simulink model "asbhl20"  (R2016b)
settings: Solver=ode3  StartTime=0.0  StopTime=61  FixedStep=1/120  RelTol=1e-3  AbsTol=1e-6
PreLoadFcn:
  | load asbhl20data.mat
InitFcn:
  | timeSince1970.Value = etime(datevec(now),[1970, 1, 1, 0, 0, 0]);
values from neighbouring files (symbols this model uses):
  maxPackets = 100    [asbhl20data.mat]
  Tc = 0.0166666666667    [asbhl20GlobalChildrenData.mat]
  x_cg = 4.78635044684    [asbhl20data.mat]
undefined symbols (not defined in the file or in its folder): m, message, Receive, s, Send, sigbuilder_block
libraries: aerolibfltsims x5, simulink x4, asbhl20GPS x2, aerolibnav x2, asbhl20env x1, asbhl20airdata x1, asbhl20ralt x1, asbhl20commsys x1, asbhl20FADEC x1, asbhl20sensors x1, asbhl20LGC x1, asbhl20vehicle x1
(part 1 of 3)
Description:
  | HL-20 auto-landing example - top level model / entry point of model
  | 
  | The HL-20 escape vehicle project for the International Space Station was
  | a fully-funded research project, designed at NASA Langley by Bruce
  | Jackson et al. Wind tunnel testing was performed on this design at
  | subsonic, supersonic, and hypersonic conditions on scale models of
  | the prototype concept.
settings Model: FPTRunName=Active  ExtModeTrigMode=oneshot  ExtModeArmWhenConnect=off  ExtModeAutoUpdateStatusClock=off  Creator=The MathWorks, Inc.  LastModifiedBy=The MathWorks, Inc.
settings SolverCC: ZeroCrossControl=DisableAll
settings DataIOCC: SaveFormat=StructureWithTime  SaveOutput=off  SignalLogging=off  SaveTime=off  StateSaveName=xbase  TimeSaveName=tsim  OutputSaveName=ysim  SignalLoggingName=sigsOut
settings OptimizationCC: BlockReduction=off  OptimizeBlockIOStorage=off  BufferReuse=off  GlobalBufferReuse=off  ExpressionFolding=off  ExpressionDepthLimit=2147483647  LocalBlockOutputs=off  InitFltsAndDblsToZero=on  EfficientFloat2IntCast=on  LifeSpan=inf
settings DebuggingCC: UnderspecifiedInitializationDetection=Classic  CheckExecutionContextPreStartOutputMsg=on  CheckExecutionContextRuntimeOutputMsg=on  MultiTaskCondExecSysMsg=none  SigSpecEnsureSampleTimeMsg=none  ParameterPrecisionLossMsg=none  FcnCallInpInsideContextMsg=warning  UniqueDataStoreMsg=error  AllowSymbolicDim=off  ModelReferenceSymbolNameMessage=none  StateNameClashWarn=warning  StrictBusMsg=ErrorOnBusTreatedAsVector  SFUnexpectedBacktrackingDiag=warning  SFNoUnconditionalDefaultTransitionDiag=warning  SFExecutionAtInitializationDiag=none
settings HardwareCC: ProdBitPerPointer=32  ProdBitPerSizeT=32  ProdBitPerPtrDiffT=32  ProdLargestAtomicFloat=None  ProdIntDivRoundTo=Undefined  ProdEndianess=Unspecified  ProdWordSize=32  ProdHWDeviceType=32-bit Generic  TargetBitPerPointer=64  TargetBitPerSizeT=64  TargetBitPerPtrDiffT=64  TargetLongLongMode=on  TargetIntDivRoundTo=Zero  TargetEndianess=LittleEndian  TargetWordSize=64  TargetHWDeviceType=MATLAB Host
settings ModelReferenceCC: UpdateModelReferenceTargets=IfOutOfDate  CheckModelReferenceTargetMessage=none  ModelReferencePassRootInputsByReference=off  PropagateSignalLabelsOutOfModel=off
settings SFSimCC: SimParseCustomCode=off
settings CodeAppCC: MaxIdLength=63
settings GRTTargetCC: TargetLangStandard=C89/C90 (ANSI)  GeneratePreprocessorConditionals=Disable all  CombineOutputUpdateFcns=off  GRTInterface=on
settings ConfigComp: CovMetricSettings=d  CovHtmlReporting=on  CovSaveCumulativeToWorkspaceVar=on  CovSaveSingleToWorkspaceVar=on  CovExternalEMLEnable=off  CovSFcnEnable=off

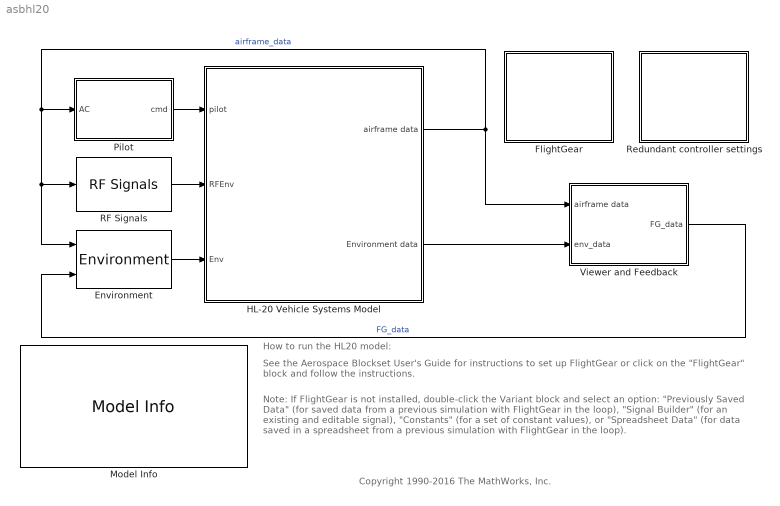
== system asbhl20 ==
  note: Copyright 1990-2016 The MathWorks, Inc.
  note: How to run the HL20 model:
  note: See the Aerospace Blockset User's Guide for instructions to set up FlightGear or click on the "FlightGear" block and follow the instructions.
  note: Note: If FlightGear is not installed, double-click the Variant block and select an option: "Previously Saved Data" (for saved data from a previous simulation with FlightGear in the loop), "Signal Builder" (for an existing and editable signal), "Constants" (for a set of constant values), or "Spreadsheet Data" (for data saved in a spreadsheet from a previous simulation with FlightGear in the loop).
  Environment : asbhl20env/Environment  SystemSampleTime=-1
  FlightGear : Subsystem  mask(FlightGear){baseFG=C:\Program Files\FlightGear\}
      mask prompts: baseFG "2. Specify FlightGear base directory"
      mask help:
      | To run this example using FlightGear locally:
      |
      | 1. Download and install FlightGear. This action opens the FlightGear download page. From this page, download and install FlightGear.
      |
      | 2. Specify FlightGear base directory.
      |
      | 3. Check FlightGear base directory. Click this button to check that FlightGear is correctly configured and installed. Upon success, the Run FlightGear block turns green and the text changes to "Start FlightGear".
      |
      | 4. Launch FlightGear for HL-20. This button installs HL-20 and runs FlightGear.
      |
      | Note: You may need administrator privilege to install HL-20.
      mask init:
      | mdl = gcs;
      | blk = gcb;
      | asbCopyAndStartFlightGear(blk,mdl,'Check','init');
      settings: AttributesFormatString=Install FlightGear
      mask Help: helpview([docroot,'/toolbox/aeroblks/aeroblks.map'],'hl20_flight_gear_help')
      mask DialogControl installFG Prompt: 1. Download and Install FlightGear
      mask DialogControl installFG Callback: web('http://flightgear.org/download/','-browser')
      mask DialogControl updateFG Prompt: 3. Check Base Directory
      mask DialogControl updateFG Callback: asbCopyAndStartFlightGear(gcb,gcs,'Check','button');
      mask DialogControl launchFG Prompt: 4. Launch HL-20 in FlightGear
      mask DialogControl launchFG Callback: asbCopyAndStartFlightGear(gcb,gcs,'CopyStart')
      mask Display: image('asbHL20FGLanding.png',[.1, .1, .8, .8],'on');
  HL-20 Vehicle Systems Model : Subsystem
      settings: RTWSystemCode=Inline
      mask Display: image('asbHL20pic.jpg')
  Model Info : simulink/Model-Wide Utilities/Model Info  BlockCM=none  Frame=on  DisplayStringWithTags=|  HorizontalTextAlignment=Center  LeftAlignmentValue=0.5  SourceBlockDiagram=asbhl20  TagMaxNumber=20
      | HL-20 Example,
      | version %<ModelVersion>
      | Aerodynamic model from 
      | Jackson E. B., Cruz C. L., 
      | "Preliminary Subsonic Aerodynamic
      | Model for Simulation Studies of the
      | HL-20 Lifting Body", 
      | NASA TM4302, August 1992.
  Pilot : Subsystem  TreatAsAtomicUnit=on
  RF Signals : asbhl20RF/RF Signals
  Redundant controller settings : Subsystem  mask(Select Redundant Controller){}
      mask help:
      | This model has a reactive controller that uses a fault-tolerant design. The controller modifies the actuator and hydraulic system as necessary. It uses a specifically designed mode logic.
      |
      | Select the implementation mode logic of the controller. The mode logic determines the actuator setup in the event of a hydraulic or actuator failure.
      |
      | Open the failure insertion panel to simulate hydraulic or actuator failures.
      |
      | Note: This feature requires a Stateflow license.
      mask init:
      | installedProducts = ver;
      | stateflowFlag = false;
      | for k=1:length(installedProducts)
      |     if strcmp(installedProducts(k).Name,'Stateflow')
      |         testLicense = license('test','stateflow');
      |         if testLicense
      |             stateflowFlag = true;
      |         end
      |     end
      | end
      | MaskObject = get_param(gcb,'MaskObject');
      | sfButtonObject = MaskObject.getDialogControl('sfLogic');
      | ssButtonObject = MaskObject.getDialogControl('ssLogic');
      | mrButtonObject = MaskObject.getDialogControl('mrLogic');
      | omButtonObject = MaskObject.getDialogControl('openModeLogic');
      | fButtonObject = MaskObject.getDialogControl('failButton');
      | if stateflowFlag
      |     sfButtonObject.Enabled = 'on';
      |     ssButtonObject.Enabled = 'on';
      |     mrButtonObject.Enabled = 'on';
      |     omButtonObject.Enabled = 'on';
      |     fButtonObject.Enabled = 'on';
      | else
      |     sfButtonObject.Enabled = 'off';
      |     ssButtonObject.Enabled = 'off';
      |     mrButtonObject.Enabled = 'off';
      |     omButtonObject.Enabled = 'off';
      |     fButtonObject.Enabled = 'off';
      | end
      | sfVar = evalin('base','Variants.FDIRApp');
      | switch sfVar
      |     case 0
      |         attStr = 'No Mode Logic';
      |     case 1
      |         attStr = 'Stateflow Chart in Subsystem';
      |     case 2
      |         attStr = 'Stateflow Chart in Model';
      |     case 3
      |         attStr = 'Stateflow Chart';
      | end
      | sfVarCheck = get_param(gcb,'AttributesFormatString');
      | if ~strcmp(sfVarCheck,attStr)
      |     set_param(gcb,'AttributesFormatString',attStr);
      | end
      settings: AttributesFormatString=No Mode Logic
      mask Help: web('http://www.mathworks.com/tagteam/21848_Mosterman Ghidella AIAA 2004 Final.pdf','-browser');
      mask DialogControl failButton Prompt: Open Failure Insertion Panel
      mask DialogControl failButton Callback: open_system(sprintf(['asbhl20/HL-20 Vehicle Systems Model/Avionics/Actuator \nSystem Failures ']),'window');
      mask DialogControl openModeLogic Prompt: Open Mode Logic
      mask DialogControl openModeLogic Callback:
      | load_system('asbhl20_FDIRApp');
      | varLogic = evalin('base','Variants.FDIRApp');
      | switch varLogic
      |     case 0
      |         open_system('asbhl20_FDIRApp/Mode Logic for Wing, Upper, and Lower/Variant Subsystem/No Logic');
      |     case 1
      |         open_system('asbhl20_FDIRApp/Mode Logic for Wing, Upper, and Lower/Variant Subsystem/Mode Logic SS/Mode Logic Chart');
      |     case 2
      |         open_system('asbhl20_FDIRApp/Mode Logic for Wing, Upper, and Lower/Variant Subsystem/Mode Logic App/Mode Logic App');
      |         open_system('asbhl20_FDIRmodelogicApp/Mode Logic');
      |     case 3
      |         open_system('asbhl20_FDIRApp/Mode Logic for Wing, Upper, and Lower/Variant Subsystem/Mode Logic Chart');
      | end
      mask DialogControl paper Prompt: Model Reuse for the Training of Fault Scenarios in Aerospace
      mask DialogControl paper Callback: web('http://www.mathworks.com/tagteam/21848_Mosterman Ghidella AIAA 2004 Final.pdf','-browser');
      mask Display: image('asbHL20ActuatorRedundancy.svg')
  Viewer and Feedback : Subsystem  Variant=on  mask(Closed Loop Variant System){}
      mask help: Select a simulation variant to identify the data source. For example, for batch mode select either a Signal Builder block or a previously saved data file. If your data source is FlightGear, run the simulation in Normal mode.
      settings: AttributesFormatString=%<ActiveVariant>
  wires:
  HL-20 Vehicle Systems Model/1(airframe data) -> Pilot/1(AC), RF Signals/1, Environment/1, Viewer and Feedback/1(airframe data)  "airframe_data"
  Pilot/1(cmd) -> HL-20 Vehicle Systems Model/1(pilot)
  Environment/1 -> HL-20 Vehicle Systems Model/3(Env)
  RF Signals/1 -> HL-20 Vehicle Systems Model/2(RFEnv)
  HL-20 Vehicle Systems Model/2(Environment data) -> Viewer and Feedback/2(env_data)
  Viewer and Feedback/1(FG_data) -> Environment/2  "FG_data"

== system asbhl20/FlightGear ==

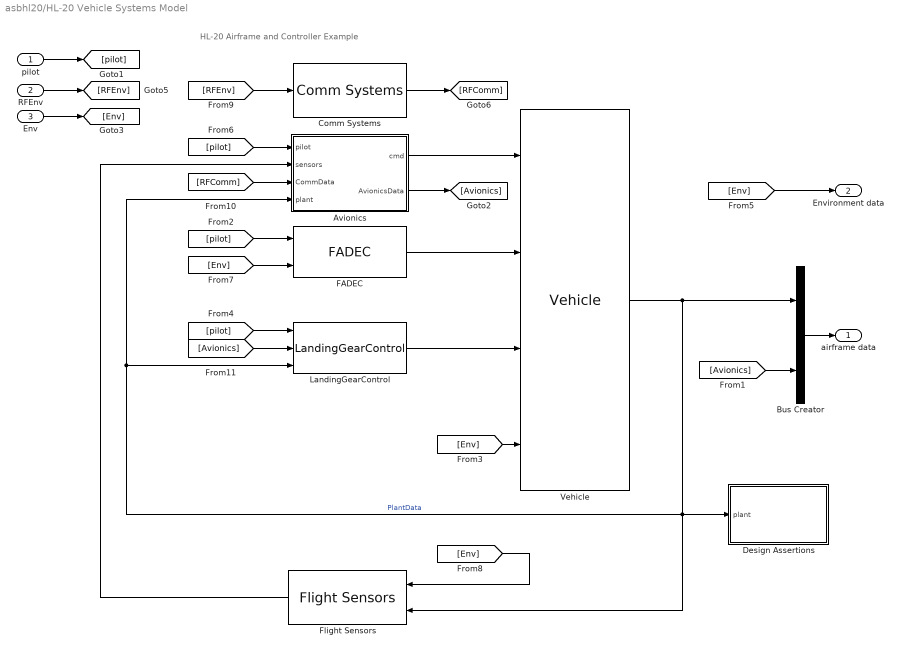
== system asbhl20/HL-20 Vehicle Systems Model ==
  note: HL-20 Airframe and Controller Example
  pilot : Inport
  RFEnv : Inport  Port=2
  Env : Inport  Port=3
  Avionics : Subsystem
  Bus Creator : BusCreator  Inputs=2
  Comm Systems : asbhl20commsys/Comm Systems
  Design Assertions : Subsystem
  FADEC : asbhl20FADEC/FADEC
  Flight Sensors : asbhl20sensors/Flight Sensors
  LandingGearControl : asbhl20LGC/LandingGearControl
  Vehicle : asbhl20vehicle/Vehicle
  airframe data : Outport
  Environment data : Outport  Port=2
  wires:
  [Env] -> Environment data/1
  [Avionics] -> LandingGearControl/2
  Avionics/1(cmd) -> Vehicle/1
  Avionics/2(AvionicsData) -> [Avionics]
  [RFComm] -> Avionics/3(CommData)
  [RFEnv] -> Comm Systems/1
  Comm Systems/1 -> [RFComm]
  [Env] -> Flight Sensors/1
  RFEnv/1 -> [RFEnv]
  Flight Sensors/1 -> Avionics/2(sensors)
  [Env] -> FADEC/2
  [pilot] -> Avionics/1(pilot)
  pilot/1 -> [pilot]
  [pilot] -> LandingGearControl/1
  [pilot] -> FADEC/1
  [Env] -> Vehicle/4
  Env/1 -> [Env]
  LandingGearControl/1 -> Vehicle/3
  FADEC/1 -> Vehicle/2
  Bus Creator/1 -> airframe data/1
  [Avionics] -> Bus Creator/2
  Vehicle/1 -> Flight Sensors/2, LandingGearControl/3, Avionics/4(plant), Design Assertions/1(plant), Bus Creator/1  "PlantData"

== system asbhl20/Pilot ==
  AC : Inport
  Bus Creator1 : BusCreator  Inputs=6
  Terminator : Terminator
  aileron : Constant  Value=0  OutDataTypeStr=single
  brake : Constant  Value=zeros(16,1)  OutDataTypeStr=single
  elevator : Constant  Value=0  OutDataTypeStr=single
  gear_handle : Constant  Value=false  OutDataTypeStr=boolean
      settings: AttributesFormatString=(false = gear up)
  rudder : Constant  Value=0  OutDataTypeStr=single
  throttle : Constant  Value=[0,0,0,0]  OutDataTypeStr=double
  cmd : Outport
  wires:
  AC/1 -> Terminator/1
  Bus Creator1/1 -> cmd/1
  rudder/1 -> Bus Creator1/3  "rudder"
  throttle/1 -> Bus Creator1/4  "throttle"
  brake/1 -> Bus Creator1/5  "brake"
  gear_handle/1 -> Bus Creator1/6  "gear_handle"
  aileron/1 -> Bus Creator1/1  "aileron"
  elevator/1 -> Bus Creator1/2  "elevator"

== system asbhl20/Redundant controller settings ==

== system asbhl20/Viewer and Feedback ==
  note: 1) Only subsystems can be added as variant choices at this level
      | 2) Blocks cannot be connected at this level as connectivity is
      | automatically determined at simulation, based on the active variant
  airframe data : Inport
  env_data : Inport  Port=2
  Constants : Subsystem  VariantControl=Variants.FlightGear == 3
  FlightGear : Subsystem  TreatAsAtomicUnit=on  VariantControl=Variants.FlightGear == 1
  Previously saved data : Subsystem  VariantControl=Variants.FlightGear == 0
  Signal Builder : Subsystem  VariantControl=Variants.FlightGear == 2
  Spreadsheet data : Subsystem  VariantControl=Variants.FlightGear == 4
  FG_data : Outport  OutDataTypeStr=Bus: FlightGearBus

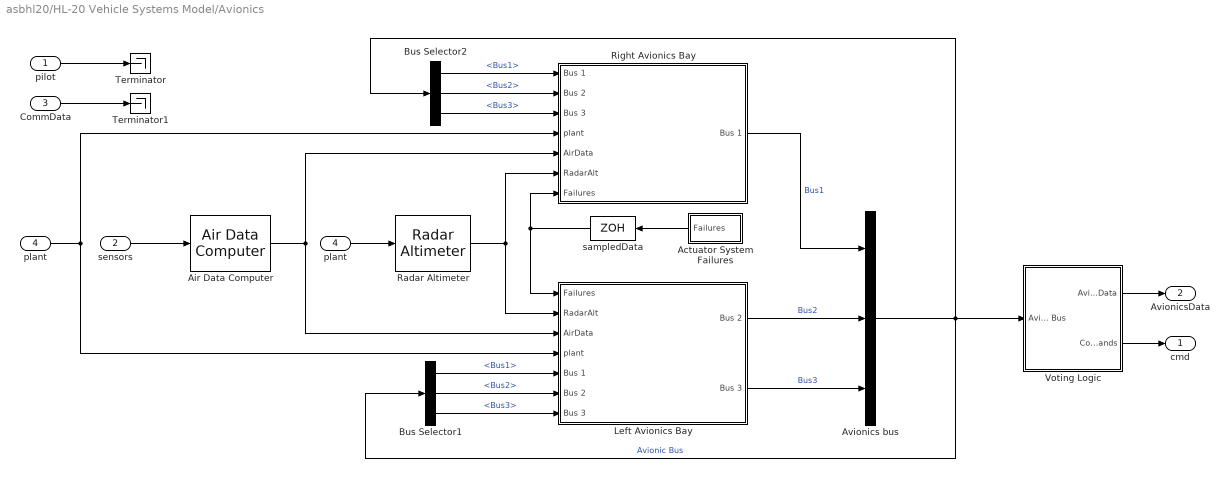
== system asbhl20/HL-20 Vehicle Systems Model/Avionics ==
  pilot : Inport
  sensors : Inport  Port=2
  CommData : Inport  Port=3
  plant : Inport  Port=4
  "Actuator System Failures " : Subsystem
  Air Data Computer : asbhl20airdata/Air Data Computer
  Avionics bus : BusCreator  Inputs=3
  Bus Selector1 : BusSelector  OutputSignals=Bus1,Bus2,Bus3
  Bus Selector2 : BusSelector  OutputSignals=Bus1,Bus2,Bus3
  Left Avionics Bay : Subsystem
  Radar Altimeter : asbhl20ralt/Radar Altimeter
  Right Avionics Bay : Subsystem
  Terminator : Terminator
  Terminator1 : Terminator
  Voting Logic : Subsystem
  "plant " : InportShadow  Port=4
  sampledData : ZeroOrderHold  SampleTime=Tc
  cmd : Outport
  AvionicsData : Outport  Port=2
  wires:
  "plant "/1 -> Radar Altimeter/1
  Radar Altimeter/1 -> Left Avionics Bay/2(RadarAlt), Right Avionics Bay/6(RadarAlt)
  CommData/1 -> Terminator1/1
  pilot/1 -> Terminator/1
  Right Avionics Bay/1(Bus 1) -> Avionics bus/1  "Bus1"
  Left Avionics Bay/1(Bus 2) -> Avionics bus/2  "Bus2"
  Avionics bus/1 -> Bus Selector1/1, Voting Logic/1(Avionic Bus), Bus Selector2/1  "Avionic Bus"
  plant/1 -> Right Avionics Bay/4(plant), Left Avionics Bay/4("plant ")
  sensors/1 -> Air Data Computer/1
  Bus Selector2/1 -> Right Avionics Bay/1("Bus 1 ")  "<Bus1>"
  Bus Selector2/2 -> Right Avionics Bay/2(Bus 2)  "<Bus2>"
  Bus Selector2/3 -> Right Avionics Bay/3(Bus 3)  "<Bus3>"
  Bus Selector1/1 -> Left Avionics Bay/5(Bus 1)  "<Bus1>"
  Bus Selector1/2 -> Left Avionics Bay/6("Bus 2 ")  "<Bus2>"
  Bus Selector1/3 -> Left Avionics Bay/7("Bus 3 ")  "<Bus3>"
  Voting Logic/1(Avionics Data) -> AvionicsData/1
  Voting Logic/2(Commands) -> cmd/1
  "Actuator System Failures "/1(Failures) -> sampledData/1
  sampledData/1 -> Right Avionics Bay/7(Failures), Left Avionics Bay/1(Failures)
  Left Avionics Bay/2(Bus 3) -> Avionics bus/3  "Bus3"
  Air Data Computer/1 -> Right Avionics Bay/5(AirData), Left Avionics Bay/3(AirData)

== system asbhl20/HL-20 Vehicle Systems Model/Design Assertions ==
  plant : Inport
  Bus Selector1 : BusSelector  OutputSignals=Mach
  Check Mach Limit : simulink/Model Verification/Check Static  Upper Bound  Description=u <= 0.92  max=0.92  max_included=on  enabled=off  stopWhenAssertionFail=on  export=off  icon=graphic
      settings: AttributesFormatString=Upper Limit = %<max>
  wires:
  plant/1 -> Bus Selector1/1
  Bus Selector1/1 -> Check Mach Limit/1  "<Mach>"

== system asbhl20/Viewer and Feedback/Constants ==
  airframe data : Inport
  env_data : Inport  Port=2
  Bus Creator1 : BusCreator  Inputs=8
  Constant : Constant
  Constant1 : Constant  Value=29.92
  Constant2 : Constant  Value=20
  Constant3 : Constant  Value=0  OutDataTypeStr=uint32
  Ground{,1..2,5} (4 alike) : Ground
  Terminator : Terminator
  Terminator1 : Terminator
  FG_data : Outport  OutDataTypeStr=Bus: FlightGearBus
  wires:
  Constant/1 -> Bus Creator1/6  "hground"
  Bus Creator1/1 -> FG_data/1
  Constant3/1 -> Bus Creator1/8  "icing"
  Constant1/1 -> Bus Creator1/5  "press_inhg"
  Constant2/1 -> Bus Creator1/4  "temp_c"
  Ground2/1 -> Bus Creator1/3  "turbulence_norm"
  Ground1/1 -> Bus Creator1/2  "wind_dir_deg"
  Ground/1 -> Bus Creator1/1  "wind_speed_kt"
  Ground5/1 -> Bus Creator1/7  "magvar"
  airframe data/1 -> Terminator/1
  env_data/1 -> Terminator1/1

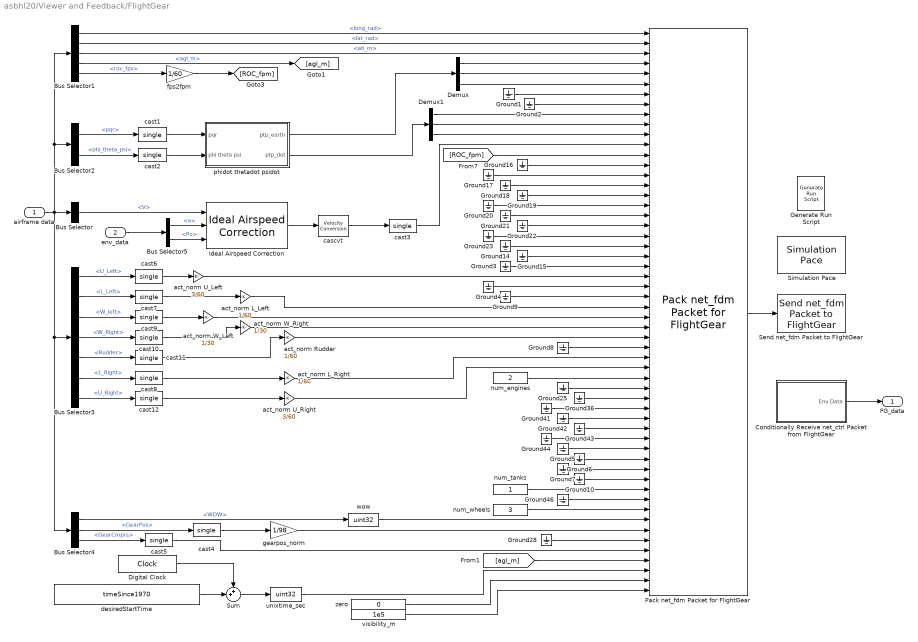
== system asbhl20/Viewer and Feedback/FlightGear ==
  airframe data : Inport  SampleTime=Tc
  env_data : Inport  Port=2  SampleTime=Tc
  Bus Selector : BusSelector  OutputSignals=PlantData.V
  Bus Selector1 : BusSelector  OutputSignals=PlantData.PosLLA.long_rad,PlantData.PosLLA.lat_rad,PlantData.PosLLA.alt_m,PlantData.PosLLA.agl_m,PlantData.PosLLA.roc_fps
  Bus Selector2 : BusSelector  OutputSignals=PlantData.pqr,PlantData.phi_theta_psi
  Bus Selector3 : BusSelector  OutputSignals=PlantData.Act_positions.U_Left,PlantData.Act_positions.L_Left,PlantData.Act_positions.W_left,PlantData.Act_positions.W_Right,PlantData.Act_positions.Rudder,PlantData.Act_positions.L_Right,PlantData.Act_positions.U_Right
  Bus Selector4 : BusSelector  OutputSignals=PlantData.LGData.WOW,PlantData.LGData.GearPos,PlantData.LGData.GearCmprs
  Bus Selector5 : BusSelector  OutputSignals=a,Po
  Conditionally Receive net_ctrl Packet from FlightGear : Subsystem
  Demux : Demux  Outputs=3
  Demux1 : Demux  Outputs=3
  Digital Clock : DigitalClock  SampleTime=Tc
  Generate Run Script : aerolibfltsims/Generate Run Script  OutputFileName=runfg.bat  FlightGearBaseDirectory=C:\Program Files\FlightGear\  GeometryModelName=HL20  DestinationPort=5502  OriginAddress=127.0.0.1  OriginPort=5505  LocalAddress=127.0.0.1  AirportId=KSFO  RunwayId=10L  InitialAltitude=7224  InitialHeading=113  OffsetDistance=4.72  OffsetAzimuth=0  GenerateFile=off  Architecture=Default  dataFlow=Send-Receive
  Ground{1..10,14..23,25,28,36,41..44,46} (28 alike) : Ground
  Ideal Airspeed Correction : aerolibasang/Ideal Airspeed Correction  units=Metric (MKS)  vel_in=TAS  vel_out_tas=CAS  vel_out_eas=CAS  vel_out_cas=TAS  action=Warning
  Pack net_fdm Packet for FlightGear : aerolibfltsims/Pack net_fdm Packet for FlightGear  FlightGearVersion=v2016.1  ShowPositionAttitudeInputs=on  ShowVelocityAccelerationInputs=on  ShowControlSurfacePositionInputs=on  ShowEngineFuelInputs=on  ShowLandingGearInputs=on  ShowEnvironmentInputs=on  SampleTime=1/30
  Send net_fdm Packet to FlightGear : aerolibfltsims/Send net_fdm Packet to FlightGear  DestinationIpAddress=127.0.0.1  DestinationPort=5502  LocalIpPort=-1  varLen=off  SampleTime=1/30
  Simulation Pace : aerolibanimutils/Simulation Pace  SimulationPace=1  SleepMode=MATLAB Thread  OutputPaceError=off  SampleTime=1/30
      settings: AttributesFormatString=%<SimulationPace> sec/sec
  Sum : Sum  Inputs=++|
  act_norm L_Left : Gain  Gain=1/60
      settings: AttributesFormatString=%<Gain>
  act_norm L_Right : Gain  Gain=1/60
      settings: AttributesFormatString=%<Gain>
  act_norm Rudder : Gain  Gain=1/60
      settings: AttributesFormatString=%<Gain>
  act_norm U_Left : Gain  Gain=3/60
      settings: AttributesFormatString=%<Gain>
  act_norm U_Right : Gain  Gain=3/60
      settings: AttributesFormatString=%<Gain>
  act_norm W_Left : Gain  Gain=1/30
      settings: AttributesFormatString=%<Gain>
  act_norm W_Right : Gain  Gain=1/30
      settings: AttributesFormatString=%<Gain>
  cascvt : aerolibconvert/Velocity Conversion  IU=m/s  OU=kts
  cast{1..12} (12 alike) : DataTypeConversion  OutDataTypeStr=single  SaturateOnIntegerOverflow=on
  desiredStartTime : Constant  Value=timeSince1970
  fps2fpm : Gain  Gain=1/60
  gearpos_norm : Gain  Gain=1/98
      settings: AttributesFormatString=%<Gain>
  num_engines : Constant  Value=2  OutDataTypeStr=uint32
  num_tanks : Constant  OutDataTypeStr=uint32
  num_wheels : Constant  Value=3  OutDataTypeStr=uint32
  phidot thetadot psidot : Subsystem
  unixtime_sec : DataTypeConversion  OutDataTypeStr=uint32  SaturateOnIntegerOverflow=on
  visibility_m : Constant  Value=1e5  OutDataTypeStr=single
  wow : DataTypeConversion  OutDataTypeStr=uint32  SaturateOnIntegerOverflow=on
  zero : Constant  Value=0  OutDataTypeStr=int32
  FG_data : Outport  OutDataTypeStr=Bus: FlightGearBus
  wires:
  Ground9/1 -> Pack net_fdm Packet for FlightGear/27
  act_norm L_Right/1 -> Pack net_fdm Packet for FlightGear/33
  Ground10/1 -> Pack net_fdm Packet for FlightGear/45
  wow/1 -> Pack net_fdm Packet for FlightGear/49
  cast11/1 -> act_norm Rudder/1
  cast10/1 -> act_norm W_Right/1
  cast9/1 -> act_norm W_Left/1
  cast8/1 -> act_norm L_Right/1
  Pack net_fdm Packet for FlightGear/1 -> Send net_fdm Packet to FlightGear/1
  Ground8/1 -> Pack net_fdm Packet for FlightGear/32
  act_norm U_Right/1 -> Pack net_fdm Packet for FlightGear/34
  act_norm Rudder/1 -> Pack net_fdm Packet for FlightGear/31
  act_norm W_Right/1 -> Pack net_fdm Packet for FlightGear/30
  act_norm W_Left/1 -> Pack net_fdm Packet for FlightGear/29
  act_norm L_Left/1 -> Pack net_fdm Packet for FlightGear/28
  Ground4/1 -> Pack net_fdm Packet for FlightGear/26
  Ground7/1 -> Pack net_fdm Packet for FlightGear/44
  Ground6/1 -> Pack net_fdm Packet for FlightGear/43
  Ground5/1 -> Pack net_fdm Packet for FlightGear/42
  Ground3/1 -> Pack net_fdm Packet for FlightGear/24
  Demux1/3 -> Pack net_fdm Packet for FlightGear/11
  Demux1/2 -> Pack net_fdm Packet for FlightGear/10
  Demux1/1 -> Pack net_fdm Packet for FlightGear/9
  Ground2/1 -> Pack net_fdm Packet for FlightGear/8
  Ground1/1 -> Pack net_fdm Packet for FlightGear/7
  act_norm U_Left/1 -> Pack net_fdm Packet for FlightGear/25
  [agl_m] -> Pack net_fdm Packet for FlightGear/53
  Bus Selector1/4 -> [agl_m]  "<agl_m>"
  Demux/3 -> Pack net_fdm Packet for FlightGear/6
  Demux/2 -> Pack net_fdm Packet for FlightGear/5
  Demux/1 -> Pack net_fdm Packet for FlightGear/4
  Bus Selector1/3 -> Pack net_fdm Packet for FlightGear/3  "<alt_m>"
  Bus Selector1/2 -> Pack net_fdm Packet for FlightGear/2  "<lat_rad>"
  Bus Selector1/1 -> Pack net_fdm Packet for FlightGear/1  "<long_rad>"
  gearpos_norm/1 -> Pack net_fdm Packet for FlightGear/50
  cast12/1 -> act_norm U_Right/1
  cast7/1 -> act_norm L_Left/1
  cast6/1 -> act_norm U_Left/1
  Bus Selector3/7 -> cast12/1  "<U_Right>"
  Bus Selector3/5 -> cast11/1  "<Rudder>"
  Bus Selector3/4 -> cast10/1  "<W_Right>"
  Bus Selector3/3 -> cast9/1  "<W_left>"
  Bus Selector3/6 -> cast8/1  "<L_Right>"
  Bus Selector3/2 -> cast7/1  "<L_Left>"
  Bus Selector3/1 -> cast6/1  "<U_Left>"
  cast5/1 -> Pack net_fdm Packet for FlightGear/52
  Bus Selector4/3 -> cast5/1  "<GearCmprs>"
  cast4/1 -> gearpos_norm/1
  Bus Selector4/2 -> cast4/1  "<GearPos>"
  fps2fpm/1 -> [ROC_fpm]
  [ROC_fpm] -> Pack net_fdm Packet for FlightGear/13
  Bus Selector5/2 -> Ideal Airspeed Correction/3  "<Po>"
  Bus Selector5/1 -> Ideal Airspeed Correction/2  "<a>"
  env_data/1 -> Bus Selector5/1
  Bus Selector4/1 -> wow/1  "<WOW>"
  Bus Selector/1 -> Ideal Airspeed Correction/1  "<V>"
  Bus Selector2/2 -> cast2/1  "<phi_theta_psi>"
  Bus Selector2/1 -> cast1/1  "<pqr>"
  phidot thetadot psidot/2(ptp_dot) -> Demux1/1
  phidot thetadot psidot/1(ptp_earth) -> Demux/1
  cast3/1 -> Pack net_fdm Packet for FlightGear/12
  cast1/1 -> phidot thetadot psidot/1(pqr)
  cast2/1 -> phidot thetadot psidot/2(phi theta psi)
  visibility_m/1 -> Pack net_fdm Packet for FlightGear/56
  zero/1 -> Pack net_fdm Packet for FlightGear/55
  unixtime_sec/1 -> Pack net_fdm Packet for FlightGear/54
  Sum/1 -> unixtime_sec/1
  desiredStartTime/1 -> Sum/2
  Digital Clock/1 -> Sum/1
  Bus Selector1/5 -> fps2fpm/1  "<roc_fps>"
  cascvt/1 -> cast3/1
  Ideal Airspeed Correction/1 -> cascvt/1
  airframe data/1 -> Bus Selector3/1, Bus Selector4/1, Bus Selector1/1, Bus Selector2/1, Bus Selector/1
  Ground28/1 -> Pack net_fdm Packet for FlightGear/51
  num_wheels/1 -> Pack net_fdm Packet for FlightGear/48
  Ground46/1 -> Pack net_fdm Packet for FlightGear/47
  num_tanks/1 -> Pack net_fdm Packet for FlightGear/46
  Ground44/1 -> Pack net_fdm Packet for FlightGear/41
  Ground43/1 -> Pack net_fdm Packet for FlightGear/40
  Ground42/1 -> Pack net_fdm Packet for FlightGear/39
  Ground41/1 -> Pack net_fdm Packet for FlightGear/38
  Ground36/1 -> Pack net_fdm Packet for FlightGear/37
  Ground25/1 -> Pack net_fdm Packet for FlightGear/36
  num_engines/1 -> Pack net_fdm Packet for FlightGear/35
  Ground15/1 -> Pack net_fdm Packet for FlightGear/23
  Ground14/1 -> Pack net_fdm Packet for FlightGear/22
  Ground23/1 -> Pack net_fdm Packet for FlightGear/21
  Ground22/1 -> Pack net_fdm Packet for FlightGear/20
  Ground21/1 -> Pack net_fdm Packet for FlightGear/19
  Ground20/1 -> Pack net_fdm Packet for FlightGear/18
  Ground19/1 -> Pack net_fdm Packet for FlightGear/17
  Ground18/1 -> Pack net_fdm Packet for FlightGear/16
  Ground17/1 -> Pack net_fdm Packet for FlightGear/15
  Ground16/1 -> Pack net_fdm Packet for FlightGear/14
  Conditionally Receive net_ctrl Packet from FlightGear/1(Env Data) -> FG_data/1

== system asbhl20/Viewer and Feedback/Previously saved data ==
  airframe data : Inport  SampleTime=Tc
  env_data : Inport  Port=2  SampleTime=Tc
  Bus Creator1 : BusCreator  Inputs=8  OutDataTypeStr=Bus: FlightGearBus
  Data Type Conversion : DataTypeConversion  OutDataTypeStr=uint32
  Demux : Demux  Outputs=8
  From File : FromFile  FileName=asbhl20FlightGear.mat  SampleTime=0
  Terminator1 : Terminator
  Terminator2 : Terminator
  FG_data : Outport  OutDataTypeStr=Bus: FlightGearBus
  wires:
  airframe data/1 -> Terminator1/1
  env_data/1 -> Terminator2/1
  From File/1 -> Demux/1
  Demux/6 -> Bus Creator1/6  "hground"
  Bus Creator1/1 -> FG_data/1
  Data Type Conversion/1 -> Bus Creator1/8  "icing"
  Demux/7 -> Bus Creator1/7  "magvar"
  Demux/4 -> Bus Creator1/4  "temp_c"
  Demux/3 -> Bus Creator1/3  "turbulence_norm"
  Demux/2 -> Bus Creator1/2  "wind_dir_deg"
  Demux/1 -> Bus Creator1/1  "wind_speed_kt"
  Demux/8 -> Data Type Conversion/1
  Demux/5 -> Bus Creator1/5  "press_inhg"

== system asbhl20/Viewer and Feedback/Signal Builder ==
  airframe data : Inport  SampleTime=Tc
  env_data : Inport  Port=2  SampleTime=Tc
  Bus Creator1 : BusCreator  Inputs=8  OutDataTypeStr=Bus: FlightGearBus
  Data Type Conversion : DataTypeConversion  OutDataTypeStr=uint32
  Signal Builder : Subsystem  Tag=STV Subsys  LoadFcn=sigbuilder_block('load');  StartFcn=sigbuilder_block('start');  StopFcn=sigbuilder_block('stop');  ClipboardFcn=sigbuilder_block('clipboard');  mask(Sigbuilder block){tuvar=[0:10]}
      mask help: Simulink:masks:SigbuilderBlock_MD
      mask init:
      | if ~strcmp(get_param(bdroot(gcbh),'SimulationStatus'),'stopped') tuvar = sigbuilder_block('maskInit'); end
      settings: CopyFcn=sigbuilder_block('copy');  DeleteFcn=sigbuilder_block('delete');  ModelCloseFcn=sigbuilder_block('modelClose');  PreSaveFcn=sigbuilder_block('preSave');  PauseFcn=sigbuilder_block('pause');  ContinueFcn=sigbuilder_block('continue');  NameChangeFcn=sigbuilder_block('namechange');  OpenFcn=sigbuilder_block('open',[229.5 6 638.25 699 ]);  CloseFcn=sigbuilder_block('close');
      mask Display: plot(0, 0, 100, 100,[2, 2, 32, 32, 2], [68, 8, 8, 68, 68],[32, 2], [38, 38], [32, 19, 2],[53, 60, 44], [32, 17, 17, 2],[16, 16, 31, 31]);txt = getActiveGroup(gcbh);text(2, 100, txt,'verticalAlignment', 'top');
  Terminator1 : Terminator
  Terminator2 : Terminator
  FG_data : Outport  OutDataTypeStr=Bus: FlightGearBus
  wires:
  env_data/1 -> Terminator2/1
  airframe data/1 -> Terminator1/1
  Signal Builder/6(hground) -> Bus Creator1/6  "hground"
  Bus Creator1/1 -> FG_data/1
  Signal Builder/8(icing) -> Data Type Conversion/1  "icing(double)"
  Signal Builder/7(magvar) -> Bus Creator1/7  "magvar"
  Signal Builder/5(press_inhg) -> Bus Creator1/5  "press_inhg"
  Signal Builder/4(temp_c) -> Bus Creator1/4  "temp_c"
  Signal Builder/3(turbulence_norm) -> Bus Creator1/3  "turbulence_norm"
  Signal Builder/2(wind_dir_deg) -> Bus Creator1/2  "wind_dir_deg"
  Signal Builder/1(wind_speed_kt) -> Bus Creator1/1  "wind_speed_kt"
  Data Type Conversion/1 -> Bus Creator1/8  "icing"

== system asbhl20/Viewer and Feedback/Spreadsheet data ==
  note: From Spreadsheet block supports the following simulation modes only: Normal, Accelerator, and Rapid Accelerator.
  airframe data : Inport  SampleTime=Tc
  env_data : Inport  Port=2  SampleTime=Tc
  Bus Creator1 : BusCreator  Inputs=8  OutDataTypeStr=Bus: FlightGearBus
  Data Type Conversion : DataTypeConversion  OutDataTypeStr=uint32
  From Spreadsheet : FromSpreadsheet  FileName=asbhl20data.xlsx  SheetName=data
  Terminator1 : Terminator
  Terminator2 : Terminator
  FG_data : Outport  OutDataTypeStr=Bus: FlightGearBus
  wires:
  airframe data/1 -> Terminator1/1
  env_data/1 -> Terminator2/1
  From Spreadsheet/6 -> Bus Creator1/6  "hground"
  Bus Creator1/1 -> FG_data/1
  From Spreadsheet/8 -> Data Type Conversion/1  "icing"
  From Spreadsheet/7 -> Bus Creator1/7  "magvar"
  From Spreadsheet/4 -> Bus Creator1/4  "temp_c"
  From Spreadsheet/3 -> Bus Creator1/3  "turbulence_norm"
  From Spreadsheet/2 -> Bus Creator1/2  "wind_dir_deg"
  From Spreadsheet/1 -> Bus Creator1/1  "wind_speed_kt"
  From Spreadsheet/5 -> Bus Creator1/5  "press_inhg"
  Data Type Conversion/1 -> Bus Creator1/8  "icing"

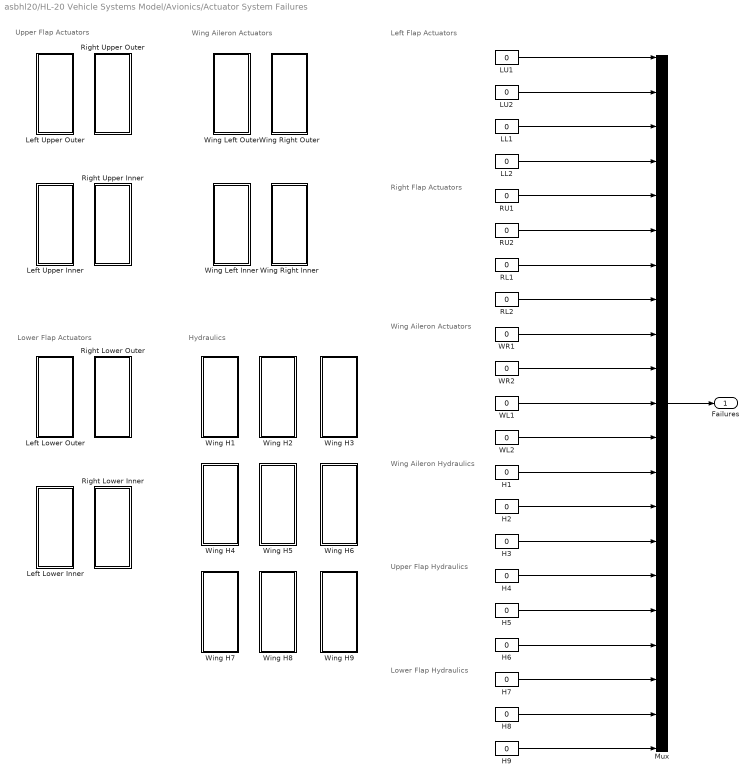
== system asbhl20/HL-20 Vehicle Systems Model/Avionics/Actuator System Failures  ==
  note: Lower Flap Hydraulics
  note: Upper Flap Hydraulics
  note: Wing Aileron Hydraulics
  note: Wing Aileron Actuators
  note: Right Flap Actuators
  note: Left Flap Actuators
  note: Hydraulics
  note: Wing Aileron Actuators
  note: Lower Flap Actuators
  note: Upper Flap Actuators
  H{1..9} (9 alike) : Constant  Value=0
  LL1 : Constant  Value=0
  LL2 : Constant  Value=0
  LU1 : Constant  Value=0
  LU2 : Constant  Value=0
  Left Lower Inner : Subsystem  DialogController=hmiCreateDDGDialog  IsWebBlock=on  mask(MathWorksWebBlock){webBlockId=1ee3efb4-48ec-42c8-9ebc-45ec9a1b45c7, webBlockType=toggleswitch, ShowInLibBrowser=on, ShowInitialText=on, HMISrcModelName=asbhl20}
      mask prompts: webBlockId "WebBlock Id"; webBlockType "WebBlock Type"; HMISrcModelName "Source Model"
      mask Help: helpview([docroot '/mapfiles/simulink.map'], 'hmi_toggle_switch')
      mask Display:
      | if strcmp(get_param(bdroot(gcb),'BlockDiagramType'), 'library')
      |     image([(matlabroot) '/toolbox/simulink/hmi/icons/ToggleSwitch.png']);
      | end
  Left Lower Outer : Subsystem  DialogController=hmiCreateDDGDialog  IsWebBlock=on  mask(MathWorksWebBlock){webBlockId=4ef0acb4-76f9-49b2-b8da-10dcd5eb02c2, webBlockType=toggleswitch, ShowInLibBrowser=on, ShowInitialText=on, HMISrcModelName=asbhl20}
      mask prompts: webBlockId "WebBlock Id"; webBlockType "WebBlock Type"; HMISrcModelName "Source Model"
      mask Help: helpview([docroot '/mapfiles/simulink.map'], 'hmi_toggle_switch')
      mask Display:
      | if strcmp(get_param(bdroot(gcb),'BlockDiagramType'), 'library')
      |     image([(matlabroot) '/toolbox/simulink/hmi/icons/ToggleSwitch.png']);
      | end
  Left Upper Inner : Subsystem  DialogController=hmiCreateDDGDialog  IsWebBlock=on  mask(MathWorksWebBlock){webBlockId=e8bd786e-071b-4c2f-ba44-9fd649cc879b, webBlockType=toggleswitch, ShowInLibBrowser=on, ShowInitialText=on, HMISrcModelName=asbhl20}
      mask prompts: webBlockId "WebBlock Id"; webBlockType "WebBlock Type"; HMISrcModelName "Source Model"
      mask Help: helpview([docroot '/mapfiles/simulink.map'], 'hmi_toggle_switch')
      mask Display:
      | if strcmp(get_param(bdroot(gcb),'BlockDiagramType'), 'library')
      |     image([(matlabroot) '/toolbox/simulink/hmi/icons/ToggleSwitch.png']);
      | end
  Left Upper Outer : Subsystem  DialogController=hmiCreateDDGDialog  IsWebBlock=on  mask(MathWorksWebBlock){webBlockId=5a508c78-52f2-4ac7-9d5f-6dd9964db8c2, webBlockType=toggleswitch, ShowInLibBrowser=on, ShowInitialText=on, HMISrcModelName=asbhl20}
      mask prompts: webBlockId "WebBlock Id"; webBlockType "WebBlock Type"; HMISrcModelName "Source Model"
      mask Help: helpview([docroot '/mapfiles/simulink.map'], 'hmi_toggle_switch')
      mask Display:
      | if strcmp(get_param(bdroot(gcb),'BlockDiagramType'), 'library')
      |     image([(matlabroot) '/toolbox/simulink/hmi/icons/ToggleSwitch.png']);
      | end
  Mux : Mux  Inputs=21
  RL1 : Constant  Value=0
  RL2 : Constant  Value=0
  RU1 : Constant  Value=0
  RU2 : Constant  Value=0
  Right Lower Inner : Subsystem  DialogController=hmiCreateDDGDialog  IsWebBlock=on  mask(MathWorksWebBlock){webBlockId=fddaa893-be99-4c15-89d8-298ebfd82649, webBlockType=toggleswitch, ShowInLibBrowser=on, ShowInitialText=on, HMISrcModelName=asbhl20}
      mask prompts: webBlockId "WebBlock Id"; webBlockType "WebBlock Type"; HMISrcModelName "Source Model"
      mask Help: helpview([docroot '/mapfiles/simulink.map'], 'hmi_toggle_switch')
      mask Display:
      | if strcmp(get_param(bdroot(gcb),'BlockDiagramType'), 'library')
      |     image([(matlabroot) '/toolbox/simulink/hmi/icons/ToggleSwitch.png']);
      | end
  Right Lower Outer : Subsystem  DialogController=hmiCreateDDGDialog  IsWebBlock=on  mask(MathWorksWebBlock){webBlockId=947d0524-d269-4a86-80e2-6750174b186a, webBlockType=toggleswitch, ShowInLibBrowser=on, ShowInitialText=on, HMISrcModelName=asbhl20}
      mask prompts: webBlockId "WebBlock Id"; webBlockType "WebBlock Type"; HMISrcModelName "Source Model"
      mask Help: helpview([docroot '/mapfiles/simulink.map'], 'hmi_toggle_switch')
      mask Display:
      | if strcmp(get_param(bdroot(gcb),'BlockDiagramType'), 'library')
      |     image([(matlabroot) '/toolbox/simulink/hmi/icons/ToggleSwitch.png']);
      | end
  Right Upper Inner : Subsystem  DialogController=hmiCreateDDGDialog  IsWebBlock=on  mask(MathWorksWebBlock){webBlockId=3005b07c-efe7-4614-badc-26d0c6fd29a3, webBlockType=toggleswitch, ShowInLibBrowser=on, ShowInitialText=on, HMISrcModelName=asbhl20}
      mask prompts: webBlockId "WebBlock Id"; webBlockType "WebBlock Type"; HMISrcModelName "Source Model"
      mask Help: helpview([docroot '/mapfiles/simulink.map'], 'hmi_toggle_switch')
      mask Display:
      | if strcmp(get_param(bdroot(gcb),'BlockDiagramType'), 'library')
      |     image([(matlabroot) '/toolbox/simulink/hmi/icons/ToggleSwitch.png']);
      | end
  Right Upper Outer : Subsystem  DialogController=hmiCreateDDGDialog  IsWebBlock=on  mask(MathWorksWebBlock){webBlockId=f7662f61-8f84-4ab6-9d59-dfc829e70c3c, webBlockType=toggleswitch, ShowInLibBrowser=on, ShowInitialText=on, HMISrcModelName=asbhl20}
      mask prompts: webBlockId "WebBlock Id"; webBlockType "WebBlock Type"; HMISrcModelName "Source Model"
      mask Help: helpview([docroot '/mapfiles/simulink.map'], 'hmi_toggle_switch')
      mask Display:
      | if strcmp(get_param(bdroot(gcb),'BlockDiagramType'), 'library')
      |     image([(matlabroot) '/toolbox/simulink/hmi/icons/ToggleSwitch.png']);
      | end
  WL1 : Constant  Value=0
  WL2 : Constant  Value=0
  WR1 : Constant  Value=0
  WR2 : Constant  Value=0
  Wing H1 : Subsystem  DialogController=hmiCreateDDGDialog  IsWebBlock=on  mask(MathWorksWebBlock){webBlockId=b7e2d375-d15c-42f0-ad23-ec92db878a8c, webBlockType=toggleswitch, ShowInLibBrowser=on, ShowInitialText=on, HMISrcModelName=asbhl20}
      mask prompts: webBlockId "WebBlock Id"; webBlockType "WebBlock Type"; HMISrcModelName "Source Model"
      mask Help: helpview([docroot '/mapfiles/simulink.map'], 'hmi_toggle_switch')
      mask Display:
      | if strcmp(get_param(bdroot(gcb),'BlockDiagramType'), 'library')
      |     image([(matlabroot) '/toolbox/simulink/hmi/icons/ToggleSwitch.png']);
      | end
  Wing H2 : Subsystem  DialogController=hmiCreateDDGDialog  IsWebBlock=on  mask(MathWorksWebBlock){webBlockId=a9134952-8b6a-4652-8026-f5b1f2b17731, webBlockType=toggleswitch, ShowInLibBrowser=on, ShowInitialText=on, HMISrcModelName=asbhl20}
      mask prompts: webBlockId "WebBlock Id"; webBlockType "WebBlock Type"; HMISrcModelName "Source Model"
      mask Help: helpview([docroot '/mapfiles/simulink.map'], 'hmi_toggle_switch')
      mask Display:
      | if strcmp(get_param(bdroot(gcb),'BlockDiagramType'), 'library')
      |     image([(matlabroot) '/toolbox/simulink/hmi/icons/ToggleSwitch.png']);
      | end
  Wing H3 : Subsystem  DialogController=hmiCreateDDGDialog  IsWebBlock=on  mask(MathWorksWebBlock){webBlockId=841f3a96-99e0-4b78-9391-e200464ec50a, webBlockType=toggleswitch, ShowInLibBrowser=on, ShowInitialText=on, HMISrcModelName=asbhl20}
      mask prompts: webBlockId "WebBlock Id"; webBlockType "WebBlock Type"; HMISrcModelName "Source Model"
      mask Help: helpview([docroot '/mapfiles/simulink.map'], 'hmi_toggle_switch')
      mask Display:
      | if strcmp(get_param(bdroot(gcb),'BlockDiagramType'), 'library')
      |     image([(matlabroot) '/toolbox/simulink/hmi/icons/ToggleSwitch.png']);
      | end
  Wing H4 : Subsystem  DialogController=hmiCreateDDGDialog  IsWebBlock=on  mask(MathWorksWebBlock){webBlockId=ea6c9873-5730-44f4-8574-cc22a9703ece, webBlockType=toggleswitch, ShowInLibBrowser=on, ShowInitialText=on, HMISrcModelName=asbhl20}
      mask prompts: webBlockId "WebBlock Id"; webBlockType "WebBlock Type"; HMISrcModelName "Source Model"
      mask Help: helpview([docroot '/mapfiles/simulink.map'], 'hmi_toggle_switch')
      mask Display:
      | if strcmp(get_param(bdroot(gcb),'BlockDiagramType'), 'library')
      |     image([(matlabroot) '/toolbox/simulink/hmi/icons/ToggleSwitch.png']);
      | end
  Wing H5 : Subsystem  DialogController=hmiCreateDDGDialog  IsWebBlock=on  mask(MathWorksWebBlock){webBlockId=308a112b-f70c-413d-a126-edf8a9e7f830, webBlockType=toggleswitch, ShowInLibBrowser=on, ShowInitialText=on, HMISrcModelName=asbhl20}
      mask prompts: webBlockId "WebBlock Id"; webBlockType "WebBlock Type"; HMISrcModelName "Source Model"
      mask Help: helpview([docroot '/mapfiles/simulink.map'], 'hmi_toggle_switch')
      mask Display:
      | if strcmp(get_param(bdroot(gcb),'BlockDiagramType'), 'library')
      |     image([(matlabroot) '/toolbox/simulink/hmi/icons/ToggleSwitch.png']);
      | end
  Wing H6 : Subsystem  DialogController=hmiCreateDDGDialog  IsWebBlock=on  mask(MathWorksWebBlock){webBlockId=6faf76e7-ead8-4cf9-8142-61c5e56a2ae8, webBlockType=toggleswitch, ShowInLibBrowser=on, ShowInitialText=on, HMISrcModelName=asbhl20}
      mask prompts: webBlockId "WebBlock Id"; webBlockType "WebBlock Type"; HMISrcModelName "Source Model"
      mask Help: helpview([docroot '/mapfiles/simulink.map'], 'hmi_toggle_switch')
      mask Display:
      | if strcmp(get_param(bdroot(gcb),'BlockDiagramType'), 'library')
      |     image([(matlabroot) '/toolbox/simulink/hmi/icons/ToggleSwitch.png']);
      | end
  Wing H7 : Subsystem  DialogController=hmiCreateDDGDialog  IsWebBlock=on  mask(MathWorksWebBlock){webBlockId=3de8ba7f-4551-46e7-8038-df0373493053, webBlockType=toggleswitch, ShowInLibBrowser=on, ShowInitialText=on, HMISrcModelName=asbhl20}
      mask prompts: webBlockId "WebBlock Id"; webBlockType "WebBlock Type"; HMISrcModelName "Source Model"
      mask Help: helpview([docroot '/mapfiles/simulink.map'], 'hmi_toggle_switch')
      mask Display:
      | if strcmp(get_param(bdroot(gcb),'BlockDiagramType'), 'library')
      |     image([(matlabroot) '/toolbox/simulink/hmi/icons/ToggleSwitch.png']);
      | end
  Wing H8 : Subsystem  DialogController=hmiCreateDDGDialog  IsWebBlock=on  mask(MathWorksWebBlock){webBlockId=10aca0c4-a92c-41e9-9d48-7082c2f0d452, webBlockType=toggleswitch, ShowInLibBrowser=on, ShowInitialText=on, HMISrcModelName=asbhl20}
      mask prompts: webBlockId "WebBlock Id"; webBlockType "WebBlock Type"; HMISrcModelName "Source Model"
      mask Help: helpview([docroot '/mapfiles/simulink.map'], 'hmi_toggle_switch')
      mask Display:
      | if strcmp(get_param(bdroot(gcb),'BlockDiagramType'), 'library')
      |     image([(matlabroot) '/toolbox/simulink/hmi/icons/ToggleSwitch.png']);
      | end
  Wing H9 : Subsystem  DialogController=hmiCreateDDGDialog  IsWebBlock=on  mask(MathWorksWebBlock){webBlockId=d72b70d1-166b-44ca-8845-65706a33c6a3, webBlockType=toggleswitch, ShowInLibBrowser=on, ShowInitialText=on, HMISrcModelName=asbhl20}
      mask prompts: webBlockId "WebBlock Id"; webBlockType "WebBlock Type"; HMISrcModelName "Source Model"
      mask Help: helpview([docroot '/mapfiles/simulink.map'], 'hmi_toggle_switch')
      mask Display:
      | if strcmp(get_param(bdroot(gcb),'BlockDiagramType'), 'library')
      |     image([(matlabroot) '/toolbox/simulink/hmi/icons/ToggleSwitch.png']);
      | end
  Wing Left Inner : Subsystem  DialogController=hmiCreateDDGDialog  IsWebBlock=on  mask(MathWorksWebBlock){webBlockId=ba272361-7e26-466f-a5dc-e685141b8821, webBlockType=toggleswitch, ShowInLibBrowser=on, ShowInitialText=on, HMISrcModelName=asbhl20}
      mask prompts: webBlockId "WebBlock Id"; webBlockType "WebBlock Type"; HMISrcModelName "Source Model"
      mask Help: helpview([docroot '/mapfiles/simulink.map'], 'hmi_toggle_switch')
      mask Display:
      | if strcmp(get_param(bdroot(gcb),'BlockDiagramType'), 'library')
      |     image([(matlabroot) '/toolbox/simulink/hmi/icons/ToggleSwitch.png']);
      | end
  Wing Left Outer : Subsystem  DialogController=hmiCreateDDGDialog  IsWebBlock=on  mask(MathWorksWebBlock){webBlockId=be983af4-910b-4a95-bbb7-cd6741bc606e, webBlockType=toggleswitch, ShowInLibBrowser=on, ShowInitialText=on, HMISrcModelName=asbhl20}
      mask prompts: webBlockId "WebBlock Id"; webBlockType "WebBlock Type"; HMISrcModelName "Source Model"
      mask Help: helpview([docroot '/mapfiles/simulink.map'], 'hmi_toggle_switch')
      mask Display:
      | if strcmp(get_param(bdroot(gcb),'BlockDiagramType'), 'library')
      |     image([(matlabroot) '/toolbox/simulink/hmi/icons/ToggleSwitch.png']);
      | end
  Wing Right Inner : Subsystem  DialogController=hmiCreateDDGDialog  IsWebBlock=on  mask(MathWorksWebBlock){webBlockId=bfcd3b2a-661c-48c5-85c3-e62e3d0a9dc8, webBlockType=toggleswitch, ShowInLibBrowser=on, ShowInitialText=on, HMISrcModelName=asbhl20}
      mask prompts: webBlockId "WebBlock Id"; webBlockType "WebBlock Type"; HMISrcModelName "Source Model"
      mask Help: helpview([docroot '/mapfiles/simulink.map'], 'hmi_toggle_switch')
      mask Display:
      | if strcmp(get_param(bdroot(gcb),'BlockDiagramType'), 'library')
      |     image([(matlabroot) '/toolbox/simulink/hmi/icons/ToggleSwitch.png']);
      | end
  Wing Right Outer : Subsystem  DialogController=hmiCreateDDGDialog  IsWebBlock=on  mask(MathWorksWebBlock){webBlockId=ad5dbfc7-fd0f-44ba-86e6-f2e3f6ce8ed6, webBlockType=toggleswitch, ShowInLibBrowser=on, ShowInitialText=on, HMISrcModelName=asbhl20}
      mask prompts: webBlockId "WebBlock Id"; webBlockType "WebBlock Type"; HMISrcModelName "Source Model"
      mask Help: helpview([docroot '/mapfiles/simulink.map'], 'hmi_toggle_switch')
      mask Display:
      | if strcmp(get_param(bdroot(gcb),'BlockDiagramType'), 'library')
      |     image([(matlabroot) '/toolbox/simulink/hmi/icons/ToggleSwitch.png']);
      | end
  Failures : Outport
  wires:
  Mux/1 -> Failures/1
  LU1/1 -> Mux/1
  LU2/1 -> Mux/2
  LL1/1 -> Mux/3
  LL2/1 -> Mux/4
  RU1/1 -> Mux/5
  RU2/1 -> Mux/6
  RL1/1 -> Mux/7
  RL2/1 -> Mux/8
  WR1/1 -> Mux/9
  WR2/1 -> Mux/10
  WL1/1 -> Mux/11
  WL2/1 -> Mux/12
  H1/1 -> Mux/13
  H2/1 -> Mux/14
  H3/1 -> Mux/15
  H5/1 -> Mux/17
  H6/1 -> Mux/18
  H7/1 -> Mux/19
  H8/1 -> Mux/20
  H9/1 -> Mux/21
  H4/1 -> Mux/16

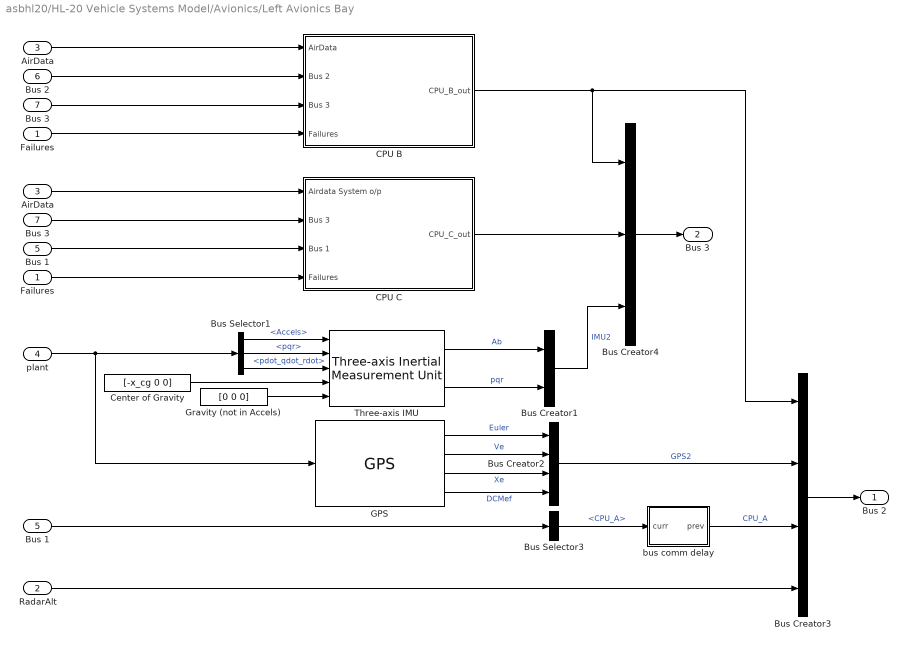
== system asbhl20/HL-20 Vehicle Systems Model/Avionics/Left Avionics Bay ==
  Failures : Inport
  RadarAlt : Inport  Port=2
  AirData : Inport  Port=3
  "plant " : Inport  Port=4
  Bus 1 : Inport  Port=5
  "Bus 2 " : Inport  Port=6
  "Bus 3 " : Inport  Port=7
  " Bus 3" : InportShadow  Port=7
  "AirData " : InportShadow  Port=3
  Bus Creator1 : BusCreator  Inputs=2
  Bus Creator2 : BusCreator  Inputs=4
  Bus Creator3 : BusCreator  Inputs=4
  Bus Creator4 : BusCreator  Inputs=3
  Bus Selector1 : BusSelector  OutputSignals=Accels,pqr,pdot_qdot_rdot
  Bus Selector3 : BusSelector  OutputSignals=CPU_A
  "Bus 1 " : InportShadow  Port=5
  CPU B : Subsystem
  CPU C : Subsystem
  Center of Gravity : Constant  Value=[-x_cg 0 0]  SampleTime=Tc
  "Failures " : InportShadow
  GPS : asbhl20GPS/GPS
  Gravity (not in Accels) : Constant  Value=[0 0 0]  SampleTime=Tc
  Three-axis IMU : aerolibnav/Three-axis Inertial Measurement Unit  units=Metric (MKS)  imu=[-x_cg 0 0]  i_Ts=Tc  dtype_a=off  w_a=190  z_a=0.707  a_sf_cc=[1 0 0; 0 1 0; 0 0 1]  a_bias=[0 0 0]  a_sat="[-inf  -inf  -inf  inf inf inf]"  dtype_g=off  w_g=190  z_g=0.707  g_sf_cc=[1 0 0; 0 1 0; 0 0 1]  g_bias=[0 0 0]  g_sens=[0 0 0]  g_sat="[-inf  -inf  -inf  inf inf inf]"  i_rand=off  i_seeds=[23093 23094 23095 23096 23097 23098]  i_pow=[0.001 0.001 0.001 0.0001 0.0001 0.0001]
  bus comm delay : Subsystem
  Bus 2 : Outport
  Bus 3 : Outport  Port=2
  wires:
  Gravity (not in Accels)/1 -> Three-axis IMU/5
  "plant "/1 -> Bus Selector1/1, GPS/1
  AirData/1 -> CPU B/1(AirData)
  CPU B/1(CPU_B_out) -> Bus Creator3/1, Bus Creator4/1
  CPU C/1(CPU_C_out) -> Bus Creator4/2
  Center of Gravity/1 -> Three-axis IMU/4
  Bus Selector1/3 -> Three-axis IMU/3  "<pdot_qdot_rdot>"
  Bus Selector1/2 -> Three-axis IMU/2  "<pqr>"
  Bus Selector1/1 -> Three-axis IMU/1  "<Accels>"
  Three-axis IMU/1 -> Bus Creator1/1  "Ab"
  Three-axis IMU/2 -> Bus Creator1/2  "pqr"
  Bus Creator1/1 -> Bus Creator4/3  "IMU2"
  Bus Creator2/1 -> Bus Creator3/2  "GPS2"
  Bus Creator3/1 -> Bus 2/1
  Bus Creator4/1 -> Bus 3/1
  Bus 1/1 -> CPU C/3(Bus 1)
  "Bus 3 "/1 -> CPU C/2(Bus 3)
  "Bus 2 "/1 -> CPU B/2(Bus 2)
  Bus Selector3/1 -> bus comm delay/1(curr)  "<CPU_A>"
  bus comm delay/1(prev) -> Bus Creator3/3  "CPU_A"
  GPS/1 -> Bus Creator2/1  "Euler"
  GPS/2 -> Bus Creator2/2  "Ve"
  RadarAlt/1 -> Bus Creator3/4
  GPS/3 -> Bus Creator2/3  "Xe"
  "AirData "/1 -> CPU C/1(Airdata System o/p)
  " Bus 3"/1 -> CPU B/3(Bus 3)
  "Bus 1 "/1 -> Bus Selector3/1
  Failures/1 -> CPU B/4(Failures)
  "Failures "/1 -> CPU C/4(Failures)
  GPS/4 -> Bus Creator2/4  "DCMef"

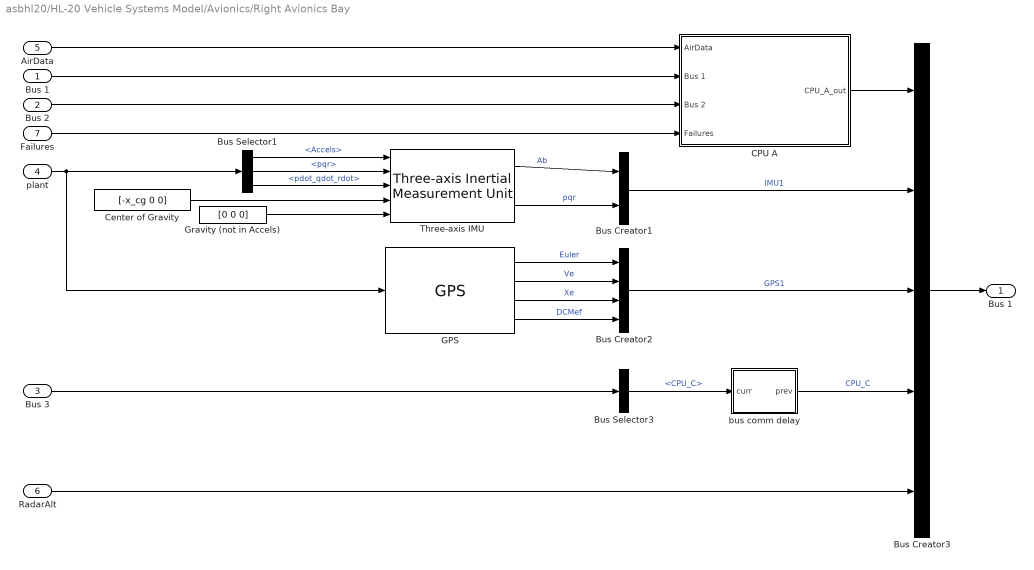
== system asbhl20/HL-20 Vehicle Systems Model/Avionics/Right Avionics Bay ==
  "Bus 1 " : Inport
  Bus 2 : Inport  Port=2
  Bus 3 : Inport  Port=3
  plant : Inport  Port=4
  AirData : Inport  Port=5
  RadarAlt : Inport  Port=6
  Failures : Inport  Port=7
  Bus Creator1 : BusCreator  Inputs=2
  Bus Creator2 : BusCreator  Inputs=4
  Bus Creator3 : BusCreator  Inputs=5
  Bus Selector1 : BusSelector  OutputSignals=Accels,pqr,pdot_qdot_rdot
  Bus Selector3 : BusSelector  OutputSignals=CPU_C
  CPU A : Subsystem
  Center of Gravity : Constant  Value=[-x_cg 0 0]  SampleTime=Tc
  GPS : asbhl20GPS/GPS
  Gravity (not in Accels) : Constant  Value=[0 0 0]  SampleTime=Tc
  Three-axis IMU : aerolibnav/Three-axis Inertial Measurement Unit  units=Metric (MKS)  imu=[-x_cg 0 0]  i_Ts=Tc  dtype_a=off  w_a=190  z_a=0.707  a_sf_cc=[1 0 0; 0 1 0; 0 0 1]  a_bias=[0 0 0]  a_sat="[-inf  -inf  -inf  inf inf inf]"  dtype_g=off  w_g=190  z_g=0.707  g_sf_cc=[1 0 0; 0 1 0; 0 0 1]  g_bias=[0 0 0]  g_sens=[0 0 0]  g_sat="[-inf  -inf  -inf  inf inf inf]"  i_rand=off  i_seeds=[23093 23094 23095 23096 23097 23098]  i_pow=[0.001 0.001 0.001 0.0001 0.0001 0.0001]
  bus comm delay : Subsystem
  Bus 1 : Outport
  wires:
  RadarAlt/1 -> Bus Creator3/5
  plant/1 -> Bus Selector1/1, GPS/1
  AirData/1 -> CPU A/1(AirData)
  Gravity (not in Accels)/1 -> Three-axis IMU/5
  Center of Gravity/1 -> Three-axis IMU/4
  Bus Selector1/3 -> Three-axis IMU/3  "<pdot_qdot_rdot>"
  Bus Selector1/2 -> Three-axis IMU/2  "<pqr>"
  Bus Selector1/1 -> Three-axis IMU/1  "<Accels>"
  Three-axis IMU/1 -> Bus Creator1/1  "Ab"
  Three-axis IMU/2 -> Bus Creator1/2  "pqr"
  Bus Creator1/1 -> Bus Creator3/2  "IMU1"
  Bus Creator2/1 -> Bus Creator3/3  "GPS1"
  CPU A/1(CPU_A_out) -> Bus Creator3/1
  Bus Creator3/1 -> Bus 1/1
  Bus 2/1 -> CPU A/3(Bus 2)
  "Bus 1 "/1 -> CPU A/2(Bus 1)
  Bus 3/1 -> Bus Selector3/1
  Bus Selector3/1 -> bus comm delay/1(curr)  "<CPU_C>"
  bus comm delay/1(prev) -> Bus Creator3/4  "CPU_C"
  GPS/1 -> Bus Creator2/1  "Euler"
  GPS/3 -> Bus Creator2/3  "Xe"
  GPS/2 -> Bus Creator2/2  "Ve"
  Failures/1 -> CPU A/4(Failures)
  GPS/4 -> Bus Creator2/4  "DCMef"
